simulink model "toy_example_es"  (R2021b)
settings: Solver=VariableStepAuto  StartTime=0.0  StopTime=50  RelTol=1e-3
libraries: slctrlblks x1
settings Model: Creator=bguo  LastModifiedBy=bguo

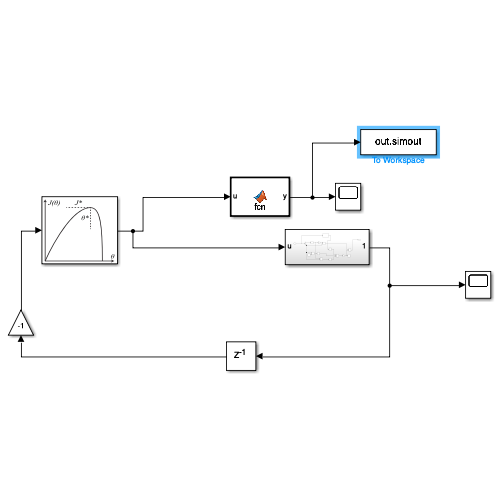
[thumbnail: Simulink's stored preview of the top-level diagram]
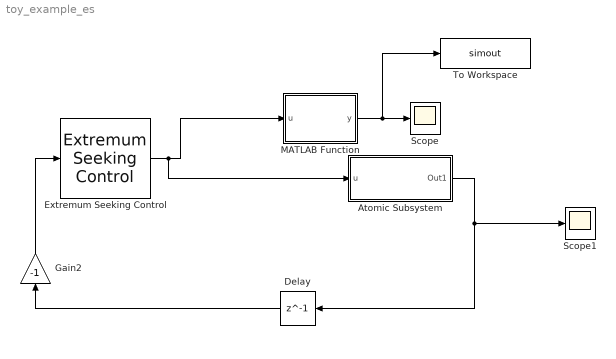
== system toy_example_es ==
  Atomic Subsystem : Subsystem
      settings: PermitHierarchicalResolution=None
  Delay : Delay  DelayLength=1  InitialCondition=0
  Extremum Seeking Control : slctrlblks/Extremum Seeking Control  timeDomainStatus=Discrete time  SampleTime=0.001  IntegratorMethods=Forward Euler  paramCount=2  initialVal=[0.9;0.9]  omega=[100;500]  gain=[15;10]  demodAmp=0.005  demodPhase=0  modAmp=0.005  modPhase=0  highPassEnable=on  highPassCutoff=30  lowPassEnable=on  lowPassCutoff=1  estimatedVarOn=off  HPFFreq=-0.97045  LPFFreq=-0.999  SampleTimeVar=0.001
      settings: SourceProductBaseCode=SD
  Gain2 : Gain  Gain=-1
  MATLAB Function : MATLAB Function  TreatAsAtomicUnit=on
  Scope : Scope
  Scope1 : Scope
  To Workspace : ToWorkspace  VariableName=simout  SaveFormat=Timeseries  SampleTime=0.01
  wires:
  Delay/1 -> Gain2/1
  Gain2/1 -> Extremum Seeking Control/1
  Extremum Seeking Control/1 -> Atomic Subsystem/1(u), MATLAB Function/1(u)
  Atomic Subsystem/1(Out1) -> Delay/1, Scope1/1
  MATLAB Function/1(y) -> To Workspace/1, Scope/1

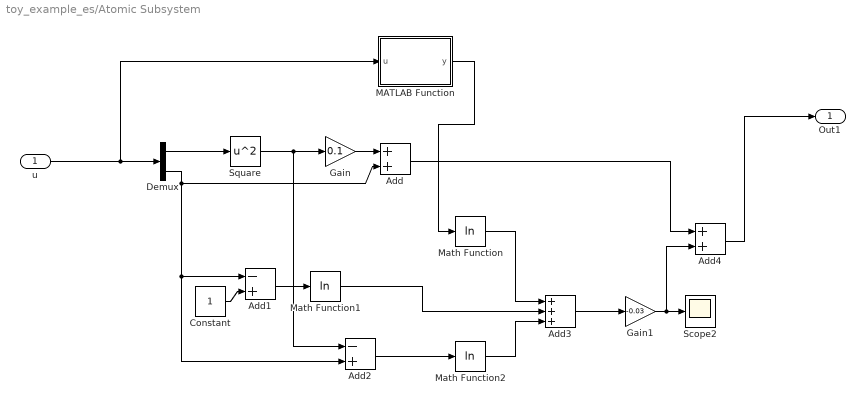
== system toy_example_es/Atomic Subsystem ==
  u : Inport
  Add : Sum
  Add1 : Sum  Inputs=-+
  Add2 : Sum  Inputs=-+
  Add3 : Sum  Inputs=+++
  Add4 : Sum
  Constant : Constant
  Demux : Demux  Outputs=2
  Gain : Gain  Gain=0.1
  Gain1 : Gain  Gain=-0.03
  MATLAB Function : MATLAB Function  TreatAsAtomicUnit=on
  Math Function : Math  Operator=log  SaturateOnIntegerOverflow=on
  Math Function1 : Math  Operator=log  SaturateOnIntegerOverflow=on
  Math Function2 : Math  Operator=log  SaturateOnIntegerOverflow=on
  Scope2 : Scope
  Square : Math  Operator=square  SaturateOnIntegerOverflow=on
  Out1 : Outport
  wires:
  Add3/1 -> Gain1/1
  Square/1 -> Add2/1, Gain/1
  Add2/1 -> Math Function2/1
  Add/1 -> Add4/1
  Math Function1/1 -> Add3/2
  Math Function2/1 -> Add3/3
  Add1/1 -> Math Function1/1
  Gain1/1 -> Add4/2, Scope2/1
  Add4/1 -> Out1/1
  u/1 -> MATLAB Function/1(u), Demux/1
  Gain/1 -> Add/1
  Demux/2 -> Add2/2, Add1/1, Add/2
  Math Function/1 -> Add3/1
  Constant/1 -> Add1/2
  Demux/1 -> Square/1
  MATLAB Function/1(y) -> Math Function/1

== matlab function toy_example_es/MATLAB Function ==
  data: u input; y output
function y = fcn(u)

y = 0.1 * (u(1))^2 + u(2);

== matlab function toy_example_es/Atomic Subsystem/MATLAB Function ==
  data: u input; y output
function y = fcn(u)

y = -0.5+(u(1)+0.5)^2+(u(2)-0.5)^2;
